simulink model "sf_aircraft_with_empty_monitor"  (R2018a)
settings: Solver=ode4  StartTime=0.0  StopTime=10  RelTol=1e-3  EnableMultiTasking=on
PreLoadFcn:
  | noise_factor=1;
  | load sf_aircraft_buses;
undefined symbols (not defined in the file or in its folder): sf_aircraft_ModeType, sigbuilder_block
libraries: simulink x21, sf_aircraft_screen_library x7, simulink_need_slupdate x2
(part 1 of 2)
settings Model: Creator=The MathWorks, Inc.  LastModifiedBy=matlab
settings DataIOCC: LimitDataPoints=on  SaveFormat=Array  ReturnWorkspaceOutputs=on  SignalLoggingName=sigsOut
settings OptimizationCC: ExpressionDepthLimit=2147483647  InitFltsAndDblsToZero=on  LifeSpan=inf
settings DebuggingCC: SaveWithParameterizedLinksMsg=none  UnderspecifiedInitializationDetection=Classic  MergeDetectMultiDrivingBlocksExec=none  CheckExecutionContextPreStartOutputMsg=on  CheckExecutionContextRuntimeOutputMsg=on  SignalResolutionControl=TryResolveAllWithWarning  MultiTaskDSMMsg=warning  MultiTaskCondExecSysMsg=none  FcnCallInpInsideContextMsg=warning  StateNameClashWarn=warning  SFUnexpectedBacktrackingDiag=warning  SFNoUnconditionalDefaultTransitionDiag=warning  SFExecutionAtInitializationDiag=none
settings HardwareCC: ProdBitPerPointer=32  ProdBitPerSizeT=32  ProdBitPerPtrDiffT=32  ProdLargestAtomicFloat=None  ProdIntDivRoundTo=Undefined  ProdEndianess=Unspecified  ProdWordSize=32  ProdHWDeviceType=32-bit Generic Real Time Simulator
settings ModelReferenceCC: PropagateSignalLabelsOutOfModel=off
settings SFSimCC: SimCustomHeaderCode="#include \"sf_aircraft_ModeType.h\""  SimParseCustomCode=off
settings RTWCC: GenCodeOnly=on  Description=Generic Real-Time Target  GenerateReport=on  CustomHeaderCode="#include \"sf_aircraft_ModeType.h\""
settings CodeAppCC: StateflowObjectComments=on
settings GRTTargetCC: TargetLangStandard=C89/C90 (ANSI)  GeneratePreprocessorConditionals=Disable all
settings ConfigComp: CovMetricSettings=dw  CovHtmlReporting=on  CovSaveCumulativeToWorkspaceVar=on  CovSaveSingleToWorkspaceVar=on  CovExternalEMLEnable=off  CovSFcnEnable=off

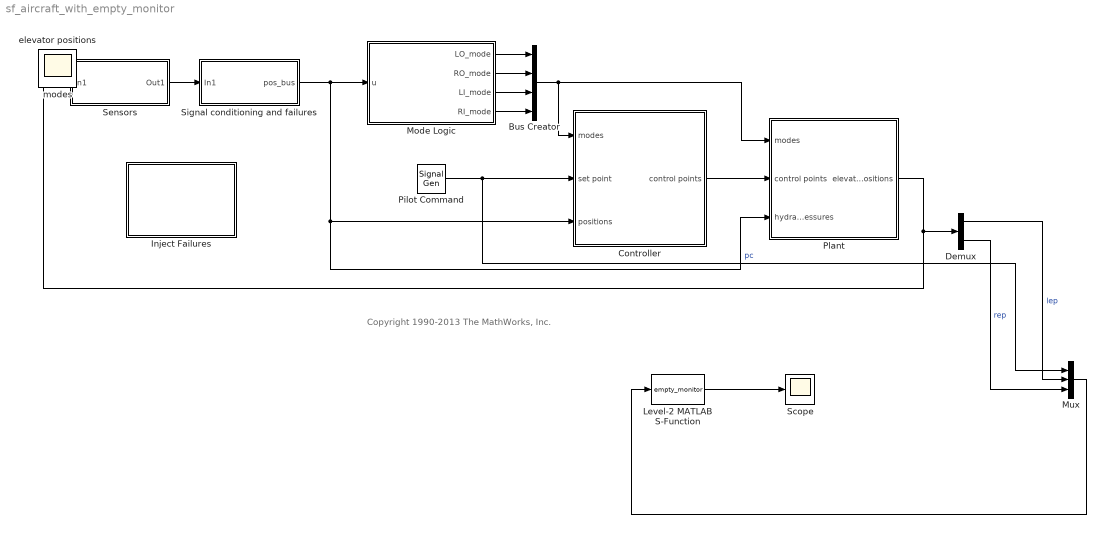
== system sf_aircraft_with_empty_monitor ==
  note: Copyright 1990-2013 The MathWorks, Inc.
  Bus Creator : BusCreator  Inputs=4
  Controller : Subsystem
  Demux : Demux  Outputs=2
  Inject Failures : Subsystem
      settings: OpenFcn=sf_aircraft_failures
      mask Display: disp('Inject Failures GUI')
  Level-2 MATLAB S-Function : M-S-Function  FunctionName=empty_monitor
  Mode Logic : Stateflow chart  TreatAsAtomicUnit=on
  Mux : Mux  Inputs=3
  Pilot Command : SignalGenerator  WaveForm=square  Frequency=0.2
  Plant : Subsystem
      mask Display: image('sf_aircraft_airplane.jpg')
  Scope : Scope
  Sensors : Subsystem
  "Signal conditioning and failures " : Subsystem
  elevator positions : Scope
  modes : Scope
  wires:
  "Signal conditioning and failures "/1(pos_bus) -> Controller/3(positions), Plant/3(hydraulic pressures), Mode Logic/1(u)
  Controller/1(control points) -> Plant/2(control points)
  Pilot Command/1 -> Mux/1, Controller/2(set point)  "pc"
  Sensors/1(Out1) -> "Signal conditioning and failures "/1(In1)
  Bus Creator/1 -> Plant/1(modes), Controller/1(modes)
  Mode Logic/1(" LO_mode") -> Bus Creator/1
  Mode Logic/2(" RO_mode") -> Bus Creator/2
  Mode Logic/3(" LI_mode") -> Bus Creator/3
  Mode Logic/4(" RI_mode") -> Bus Creator/4
  Plant/1(elevator positions) -> Demux/1, Sensors/1(In1)
  Demux/1 -> Mux/2  "lep"
  Demux/2 -> Mux/3  "rep"
  Mux/1 -> Level-2 MATLAB S-Function/1
  Level-2 MATLAB S-Function/1 -> Scope/1

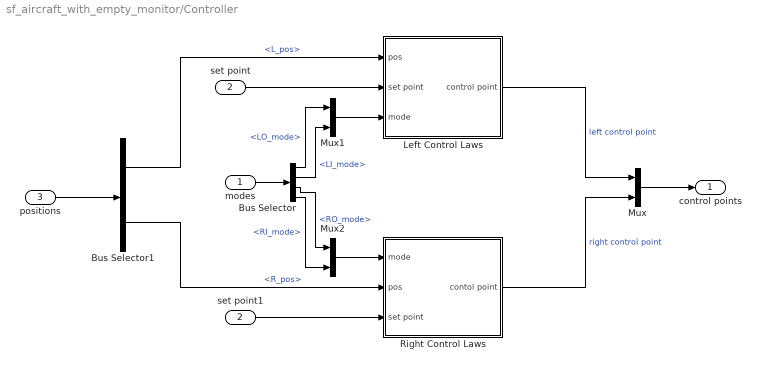
== system sf_aircraft_with_empty_monitor/Controller ==
  modes : Inport
  set point : Inport  Port=2  SampleTime=0.01
  positions : Inport  Port=3  SampleTime=0.01
  Bus Selector : BusSelector  OutputSignals=LO_mode,LI_mode,RO_mode,RI_mode
  Bus Selector1 : BusSelector  OutputSignals=L_pos,R_pos
  Left Control Laws : Subsystem
  Mux : Mux  Inputs=2
  Mux1 : Mux  Inputs=2
  Mux2 : Mux  Inputs=2
  Right Control Laws : Subsystem
  set point1 : InportShadow  Port=2  SampleTime=0.01
  control points : Outport
  wires:
  Mux/1 -> control points/1
  modes/1 -> Bus Selector/1
  Right Control Laws/1(contol point) -> Mux/2  "right control point"
  set point1/1 -> Right Control Laws/3(set point)
  Left Control Laws/1(control point) -> Mux/1  "left control point"
  set point/1 -> Left Control Laws/2(set point)
  Bus Selector/4 -> Mux2/2  "<RI_mode>"
  Bus Selector/3 -> Mux2/1  "<RO_mode>"
  Bus Selector/1 -> Mux1/1  "<LO_mode>"
  Bus Selector/2 -> Mux1/2  "<LI_mode>"
  Mux1/1 -> Left Control Laws/3(mode)
  Mux2/1 -> Right Control Laws/1(mode)
  positions/1 -> Bus Selector1/1
  Bus Selector1/1 -> Left Control Laws/1(pos)  "<L_pos>"
  Bus Selector1/2 -> Right Control Laws/2(pos)  "<R_pos>"

== system sf_aircraft_with_empty_monitor/Inject Failures ==

== system sf_aircraft_with_empty_monitor/Plant ==
  modes : Inport
  control points : Inport  Port=2  SampleTime=0.01
  hydraulic pressures : Inport  Port=3  SampleTime=0.01
  Actuators : Subsystem
  Left Elevator : Subsystem
  Mux : Mux  Inputs=2
  Mux1 : Mux  Inputs=2
  Right Elevator : Subsystem
  elevator positions : Outport
  wires:
  Mux1/1 -> elevator positions/1
  Right Elevator/2(elevator position) -> Mux1/2
  Left Elevator/1(elevator position) -> Mux1/1
  Mux/1 -> Actuators/4(piston velocity)
  Right Elevator/1(elevator velocity) -> Mux/2
  Left Elevator/2(elevator velocity) -> Mux/1
  modes/1 -> Actuators/3(modes)
  Actuators/2(Right piston force) -> Right Elevator/1(piston force)
  hydraulic pressures/1 -> Actuators/2(hydraulic pressure)
  control points/1 -> Actuators/1(control point)
  Actuators/1(Left piston force) -> Left Elevator/1(piston force)

== system sf_aircraft_with_empty_monitor/Sensors ==
  In1 : Inport
  Demux : Demux  Outputs=2
  Measured Left Inner Actuator positions : Subsystem
  Measured Left Outer Actuator positions : Subsystem
  Measured Right Inner Actuator positions : Subsystem
  Measured Right Outer Actuator positions : Subsystem
  Mux : Mux
  Out1 : Outport
  wires:
  Demux/1 -> Measured Left Inner Actuator positions/1(In1), Measured Left Outer Actuator positions/1(In1)
  Demux/2 -> Measured Right Inner Actuator positions/1(In1), Measured Right Outer Actuator positions/1(In1)
  Measured Left Outer Actuator positions/1(Out) -> Mux/1
  Measured Left Inner Actuator positions/1(Out) -> Mux/2
  Measured Right Inner Actuator positions/1(Out) -> Mux/3
  Measured Right Outer Actuator positions/1(Out) -> Mux/4
  In1/1 -> Demux/1
  Mux/1 -> Out1/1

== system sf_aircraft_with_empty_monitor/Signal conditioning and failures  ==
  note: These could be 2/4 separate processors, and typically are not residing on the PFCUs
  In1 : Inport
  Actuator Positions : Subsystem
  Bus Creator1 : BusCreator  Inputs=8  OutDataTypeStr=Bus: PositionBus  NonVirtualBus=on
  Demux : Demux
  Hydraulic Pressures : Subsystem
  pos_bus : Outport
  wires:
  Bus Creator1/1 -> pos_bus/1
  Actuator Positions/2(L_pos_fail) -> Bus Creator1/2  "L_pos_fail"
  Actuator Positions/3(R_pos) -> Bus Creator1/3  "R_pos"
  Actuator Positions/4(R_pos_fail) -> Bus Creator1/4  "R_pos_fail"
  In1/1 -> Demux/1
  Demux/1 -> Actuator Positions/1(Left Outer)
  Demux/2 -> Actuator Positions/2(Left Inner)
  Actuator Positions/1(L_pos) -> Bus Creator1/1  "L_pos"
  Demux/3 -> Actuator Positions/3(Right Inner)
  Demux/4 -> Actuator Positions/4(Right Outer)
  Hydraulic Pressures/1(H1_press) -> Bus Creator1/5  "H1_press"
  Hydraulic Pressures/2(H2_press) -> Bus Creator1/6  "H2_press"
  Hydraulic Pressures/3(H3_press) -> Bus Creator1/7  "H3_press"
  Hydraulic Pressures/4(low_press) -> Bus Creator1/8  "low_press"

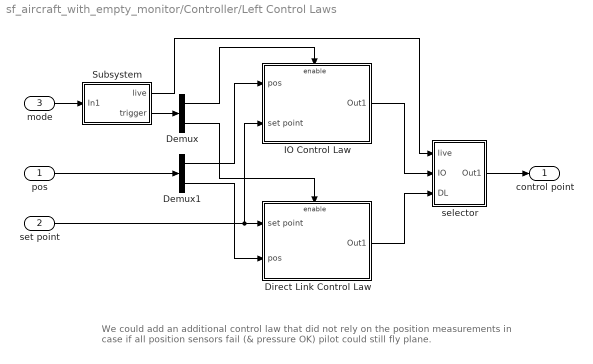
== system sf_aircraft_with_empty_monitor/Controller/Left Control Laws ==
  note: We could add an additional control law that did not rely on the position measurements
      | in case if all position sensors fail (& pressure OK) pilot could still fly plane.
  pos : Inport
  set point : Inport  Port=2  SampleTime=0.01
  mode : Inport  Port=3
  Demux : Demux  Outputs=2
  Demux1 : Demux  Outputs=2
  Direct Link Control Law : Subsystem
  IO Control Law : Subsystem
  Subsystem : Subsystem
  selector : Subsystem
  control point : Outport
  wires:
  Subsystem/1(live) -> selector/1(live)
  set point/1 -> IO Control Law/2(set point), Direct Link Control Law/1(set point)
  pos/1 -> Demux1/1
  selector/1(Out1) -> control point/1
  Direct Link Control Law/1(Out1) -> selector/3(DL)
  IO Control Law/1(Out1) -> selector/2(IO)
  Demux/2 -> Direct Link Control Law/Enable
  Demux/1 -> IO Control Law/Enable
  Subsystem/2(trigger) -> Demux/1
  mode/1 -> Subsystem/1(In1)
  Demux1/1 -> IO Control Law/1(pos)
  Demux1/2 -> Direct Link Control Law/2(pos)

== system sf_aircraft_with_empty_monitor/Controller/Right Control Laws ==
  note: We could add an additional control law that did not have to rely on the position measurements
      | in case if all position sensors fail (& pressure OK) pilot could still fly plane.
  mode : Inport
  pos : Inport  Port=2
  set point : Inport  Port=3  SampleTime=0.01
  Demux : Demux  Outputs=2
  Demux1 : Demux  Outputs=2
  Direct Link Control Law : Subsystem
  IO Control Law : Subsystem
  Subsystem : Subsystem
  selector : Subsystem
  contol point : Outport
  wires:
  selector/1(Out1) -> contol point/1
  Subsystem/1(live) -> selector/1(live)
  Demux1/1 -> IO Control Law/1(pos)
  Demux1/2 -> Direct Link Control Law/2(pos)
  set point/1 -> IO Control Law/2(set point), Direct Link Control Law/1(set point)
  pos/1 -> Demux1/1
  Direct Link Control Law/1(Out1) -> selector/3(DL)
  IO Control Law/1(Out1) -> selector/2(IO)
  Demux/2 -> Direct Link Control Law/Enable
  Demux/1 -> IO Control Law/Enable
  Subsystem/2(trigger) -> Demux/1
  mode/1 -> Subsystem/1(In1)

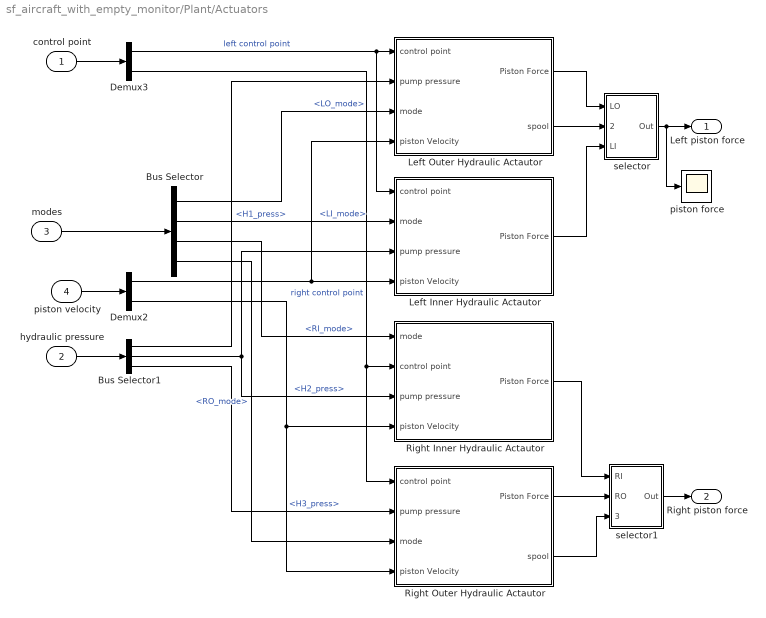
== system sf_aircraft_with_empty_monitor/Plant/Actuators ==
  control point : Inport
  hydraulic pressure : Inport  Port=2
  modes : Inport  Port=3
  piston velocity : Inport  Port=4
  Bus Selector : BusSelector  OutputSignals=LO_mode,LI_mode,RI_mode,RO_mode
  Bus Selector1 : BusSelector  OutputSignals=H1_press,H2_press,H3_press
  Demux2 : Demux  Outputs=2
  Demux3 : Demux  Outputs=2
  Left Inner Hydraulic Actautor : Subsystem
  Left Outer Hydraulic Actautor : Subsystem
  Right Inner Hydraulic Actautor : Subsystem
  Right Outer Hydraulic Actautor : Subsystem
  piston force : Scope
  selector : Subsystem
  selector1 : Subsystem
  Left piston force : Outport
  Right piston force : Outport  Port=2
  wires:
  Right Outer Hydraulic Actautor/2(spool) -> selector1/3(spool)
  Left Outer Hydraulic Actautor/2(spool) -> selector/2(spool)
  Demux3/2 -> Right Outer Hydraulic Actautor/1(control point), Right Inner Hydraulic Actautor/2(control point)  "right control point"
  control point/1 -> Demux3/1
  piston velocity/1 -> Demux2/1
  Demux2/2 -> Right Outer Hydraulic Actautor/4(piston Velocity), Right Inner Hydraulic Actautor/4(piston Velocity)
  modes/1 -> Bus Selector/1
  Bus Selector1/3 -> Right Outer Hydraulic Actautor/2(pump pressure)  "<H3_press>"
  Bus Selector1/2 -> Right Inner Hydraulic Actautor/3(pump pressure), Left Inner Hydraulic Actautor/3(pump pressure)  "<H2_press>"
  selector1/1(Out) -> Right piston force/1
  selector/1(Out) -> Left piston force/1, piston force/1
  Left Inner Hydraulic Actautor/1(Piston Force) -> selector/3(LI)
  Left Outer Hydraulic Actautor/1(Piston Force) -> selector/1(LO)
  Right Outer Hydraulic Actautor/1(Piston Force) -> selector1/2(RO)
  Right Inner Hydraulic Actautor/1(Piston Force) -> selector1/1(RI)
  Demux2/1 -> Left Outer Hydraulic Actautor/4(piston Velocity), Left Inner Hydraulic Actautor/4(piston Velocity)
  Demux3/1 -> Left Inner Hydraulic Actautor/1(control point), Left Outer Hydraulic Actautor/1(control point)  "left control point"
  Bus Selector1/1 -> Left Outer Hydraulic Actautor/2(pump pressure)  "<H1_press>"
  Bus Selector/1 -> Left Outer Hydraulic Actautor/3(mode)  "<LO_mode>"
  Bus Selector/2 -> Left Inner Hydraulic Actautor/2(mode)  "<LI_mode>"
  Bus Selector/3 -> Right Inner Hydraulic Actautor/1(mode)  "<RI_mode>"
  Bus Selector/4 -> Right Outer Hydraulic Actautor/3(mode)  "<RO_mode>"
  hydraulic pressure/1 -> Bus Selector1/1

== system sf_aircraft_with_empty_monitor/Plant/Left Elevator ==
  piston force : Inport
  Sum1 : Sum  Inputs=-+-  SaturateOnIntegerOverflow=on
  elevator Mass : Integrator
  integrator : Integrator
  viscous friction : Gain  Gain=10  SaturateOnIntegerOverflow=on  OutDataTypeStr=Inherit: Same as input  ParamDataTypeStr=Inherit: Same as input
  wind load : Gain  Gain=1000  SaturateOnIntegerOverflow=on  OutDataTypeStr=Inherit: Same as input  ParamDataTypeStr=Inherit: Same as input
  elevator position : Outport
  elevator velocity : Outport  Port=2
  wires:
  Sum1/1 -> elevator Mass/1
  elevator Mass/1 -> viscous friction/1, elevator velocity/1, integrator/1
  integrator/1 -> elevator position/1, wind load/1
  piston force/1 -> Sum1/2
  viscous friction/1 -> Sum1/3
  wind load/1 -> Sum1/1

== system sf_aircraft_with_empty_monitor/Plant/Right Elevator ==
  piston force : Inport
  Sum1 : Sum  Inputs=-+-  SaturateOnIntegerOverflow=on
  elevator Mass : Integrator
  integrator : Integrator
  viscous friction : Gain  Gain=10  SaturateOnIntegerOverflow=on  OutDataTypeStr=Inherit: Same as input  ParamDataTypeStr=Inherit: Same as input
  wind load : Gain  Gain=1000  SaturateOnIntegerOverflow=on  OutDataTypeStr=Inherit: Same as input  ParamDataTypeStr=Inherit: Same as input
  elevator velocity : Outport
  elevator position : Outport  Port=2
  wires:
  integrator/1 -> elevator position/1, wind load/1
  elevator Mass/1 -> integrator/1, viscous friction/1, elevator velocity/1
  Sum1/1 -> elevator Mass/1
  wind load/1 -> Sum1/1
  viscous friction/1 -> Sum1/3
  piston force/1 -> Sum1/2

== system sf_aircraft_with_empty_monitor/Sensors/Measured Left Inner Actuator positions ==
  In1 : Inport
  LI_pos_fail : Constant  Value=0  OutDataTypeStr=boolean
  Measured Position1 : Subsystem
  Measured Position2 : Subsystem
  Measured Position3 : Subsystem
  Mux : Mux  Inputs=3
  Outlier/failure : Subsystem  Tag=STV Subsys  LoadFcn=sigbuilder_block('load');  StartFcn=sigbuilder_block('start');  StopFcn=sigbuilder_block('stop');  ClipboardFcn=sigbuilder_block('clipboard');  mask(Sigbuilder block){tuvar=[0:10]}
      mask help: Sigbuilder GUI
      mask init:
      | if ~strcmp(get_param(bdroot,'SimulationStatus'),'stopped') tuvar = sigbuilder_block('maskInit'); end
      settings: CopyFcn=sigbuilder_block('copy');  DeleteFcn=sigbuilder_block('delete');  ModelCloseFcn=sigbuilder_block('modelClose');  PreSaveFcn=sigbuilder_block('preSave');  PauseFcn=sigbuilder_block('pause')  ContinueFcn=sigbuilder_block('continue')  NameChangeFcn=sigbuilder_block('namechange');  OpenFcn=sigbuilder_block('open',[81 97.5 519.75 399.75 ]);  CloseFcn=sigbuilder_block('close');
      mask Display: plot(0, 0, 100, 100,[2, 2, 32, 32, 2], [68, 8, 8, 68, 68],[32, 2], [38, 38], [32, 19, 2],[53, 60, 44], [32, 17, 17, 2],[16, 16, 31, 31]);txt = getActiveGroup(gcbh);text(2, 100, txt,'verticalAlignment', 'top');
  Switch : Switch  Criteria=u2 ~= 0  SaturateOnIntegerOverflow=on
  Zero-Order Hold : ZeroOrderHold  SampleTime=0.01
  Out : Outport
  wires:
  Switch/1 -> Zero-Order Hold/1
  Measured Position1/1(Out1) -> Mux/1
  Measured Position2/1(Out1) -> Mux/2
  Mux/1 -> Out/1
  Measured Position3/1(Out1) -> Mux/3
  Outlier/failure/1(Signal 1) -> Switch/1
  LI_pos_fail/1 -> Switch/2
  In1/1 -> Switch/3
  Zero-Order Hold/1 -> Measured Position3/1(position), Measured Position1/1(position), Measured Position2/1(position)

== system sf_aircraft_with_empty_monitor/Sensors/Measured Left Outer Actuator positions ==
  In1 : Inport
  LO_pos_fail : Constant  Value=0  OutDataTypeStr=boolean
  Measured Position1 : Subsystem
  Measured Position2 : Subsystem
  Measured Position3 : Subsystem
  Mux : Mux  Inputs=3
  Outlier/failure : Subsystem  Tag=STV Subsys  LoadFcn=sigbuilder_block('load');  StartFcn=sigbuilder_block('start');  StopFcn=sigbuilder_block('stop');  ClipboardFcn=sigbuilder_block('clipboard');  mask(Sigbuilder block){tuvar=[0:10]}
      mask help: Sigbuilder GUI
      mask init:
      | if ~strcmp(get_param(bdroot,'SimulationStatus'),'stopped') tuvar = sigbuilder_block('maskInit'); end
      settings: CopyFcn=sigbuilder_block('copy');  DeleteFcn=sigbuilder_block('delete');  ModelCloseFcn=sigbuilder_block('modelClose');  PreSaveFcn=sigbuilder_block('preSave');  PauseFcn=sigbuilder_block('pause')  ContinueFcn=sigbuilder_block('continue')  NameChangeFcn=sigbuilder_block('namechange');  OpenFcn=sigbuilder_block('open',[81 97.5 519.75 399.75 ]);  CloseFcn=sigbuilder_block('close');
      mask Display: plot(0, 0, 100, 100,[2, 2, 32, 32, 2], [68, 8, 8, 68, 68],[32, 2], [38, 38], [32, 19, 2],[53, 60, 44], [32, 17, 17, 2],[16, 16, 31, 31]);txt = getActiveGroup(gcbh);text(2, 100, txt,'verticalAlignment', 'top');
  Switch : Switch  Criteria=u2 ~= 0  SaturateOnIntegerOverflow=on
  Zero-Order Hold : ZeroOrderHold  SampleTime=0.01
  Out : Outport
  wires:
  Measured Position3/1(Out1) -> Mux/3
  Mux/1 -> Out/1
  Measured Position2/1(Out1) -> Mux/2
  Measured Position1/1(Out1) -> Mux/1
  Switch/1 -> Zero-Order Hold/1
  Outlier/failure/1(Signal 1) -> Switch/1
  LO_pos_fail/1 -> Switch/2
  In1/1 -> Switch/3
  Zero-Order Hold/1 -> Measured Position2/1(position), Measured Position1/1(position), Measured Position3/1(position)

== system sf_aircraft_with_empty_monitor/Sensors/Measured Right Inner Actuator positions ==
  In1 : Inport
  Measured Position1 : Subsystem
  Measured Position2 : Subsystem
  Measured Position3 : Subsystem
  Mux : Mux  Inputs=3
  Outlier/failure : Subsystem  Tag=STV Subsys  LoadFcn=sigbuilder_block('load');  StartFcn=sigbuilder_block('start');  StopFcn=sigbuilder_block('stop');  ClipboardFcn=sigbuilder_block('clipboard');  mask(Sigbuilder block){tuvar=[0:10]}
      mask help: Sigbuilder GUI
      mask init:
      | if ~strcmp(get_param(bdroot,'SimulationStatus'),'stopped') tuvar = sigbuilder_block('maskInit'); end
      settings: CopyFcn=sigbuilder_block('copy');  DeleteFcn=sigbuilder_block('delete');  ModelCloseFcn=sigbuilder_block('modelClose');  PreSaveFcn=sigbuilder_block('preSave');  PauseFcn=sigbuilder_block('pause')  ContinueFcn=sigbuilder_block('continue')  NameChangeFcn=sigbuilder_block('namechange');  OpenFcn=sigbuilder_block('open',[81 97.5 519.75 399.75 ]);  CloseFcn=sigbuilder_block('close');
      mask Display: plot(0, 0, 100, 100,[2, 2, 32, 32, 2], [68, 8, 8, 68, 68],[32, 2], [38, 38], [32, 19, 2],[53, 60, 44], [32, 17, 17, 2],[16, 16, 31, 31]);txt = getActiveGroup(gcbh);text(2, 100, txt,'verticalAlignment', 'top');
  RI_pos_fail : Constant  Value=0  OutDataTypeStr=boolean
  Switch : Switch  Criteria=u2 ~= 0  SaturateOnIntegerOverflow=on
  Zero-Order Hold : ZeroOrderHold  SampleTime=0.01
  Out : Outport
  wires:
  Switch/1 -> Zero-Order Hold/1
  Measured Position1/1(Out1) -> Mux/1
  Measured Position2/1(Out1) -> Mux/2
  Mux/1 -> Out/1
  Measured Position3/1(Out1) -> Mux/3
  Outlier/failure/1(Signal 1) -> Switch/1
  RI_pos_fail/1 -> Switch/2
  In1/1 -> Switch/3
  Zero-Order Hold/1 -> Measured Position3/1(position), Measured Position1/1(position), Measured Position2/1(position)

== system sf_aircraft_with_empty_monitor/Sensors/Measured Right Outer Actuator positions ==
  In1 : Inport
  Measured Position1 : Subsystem
  Measured Position2 : Subsystem
  Measured Position3 : Subsystem
  Mux : Mux  Inputs=3
  Outlier/failure : Subsystem  Tag=STV Subsys  LoadFcn=sigbuilder_block('load');  StartFcn=sigbuilder_block('start');  StopFcn=sigbuilder_block('stop');  ClipboardFcn=sigbuilder_block('clipboard');  mask(Sigbuilder block){tuvar=[0:10]}
      mask help: Sigbuilder GUI
      mask init:
      | if ~strcmp(get_param(bdroot,'SimulationStatus'),'stopped') tuvar = sigbuilder_block('maskInit'); end
      settings: CopyFcn=sigbuilder_block('copy');  DeleteFcn=sigbuilder_block('delete');  ModelCloseFcn=sigbuilder_block('modelClose');  PreSaveFcn=sigbuilder_block('preSave');  PauseFcn=sigbuilder_block('pause')  ContinueFcn=sigbuilder_block('continue')  NameChangeFcn=sigbuilder_block('namechange');  OpenFcn=sigbuilder_block('open',[81 97.5 519.75 399.75 ]);  CloseFcn=sigbuilder_block('close');
      mask Display: plot(0, 0, 100, 100,[2, 2, 32, 32, 2], [68, 8, 8, 68, 68],[32, 2], [38, 38], [32, 19, 2],[53, 60, 44], [32, 17, 17, 2],[16, 16, 31, 31]);txt = getActiveGroup(gcbh);text(2, 100, txt,'verticalAlignment', 'top');
  RO_pos_fail : Constant  Value=0  OutDataTypeStr=boolean
  Switch : Switch  Criteria=u2 ~= 0  SaturateOnIntegerOverflow=on
  Zero-Order Hold : ZeroOrderHold  SampleTime=0.01
  Out : Outport
  wires:
  Zero-Order Hold/1 -> Measured Position2/1(position), Measured Position1/1(position), Measured Position3/1(position)
  In1/1 -> Switch/3
  RO_pos_fail/1 -> Switch/2
  Outlier/failure/1(Signal 1) -> Switch/1
  Measured Position3/1(Out1) -> Mux/3
  Mux/1 -> Out/1
  Measured Position2/1(Out1) -> Mux/2
  Measured Position1/1(Out1) -> Mux/1
  Switch/1 -> Zero-Order Hold/1

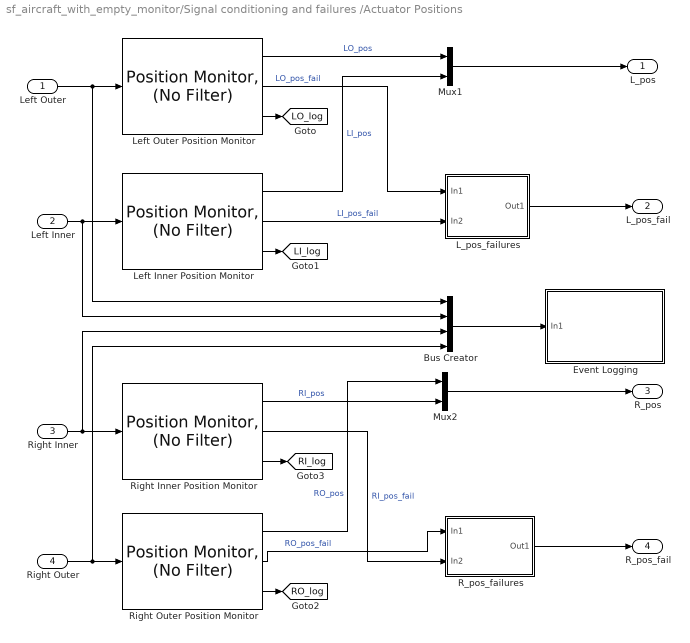
== system sf_aircraft_with_empty_monitor/Signal conditioning and failures /Actuator Positions ==
  Left Outer : Inport
  Left Inner : Inport  Port=2
  Right Inner : Inport  Port=3
  Right Outer : Inport  Port=4
  Bus Creator : BusCreator  Inputs=4
  Event Logging : Subsystem
  L_pos_failures : Subsystem
  Left Inner Position Monitor : sf_aircraft_screen_library/Position Monitor, (No Filter)
      settings: SourceProductName=Stateflow  SourceProductBaseCode=SF
  Left Outer Position Monitor : sf_aircraft_screen_library/Position Monitor, (No Filter)
      settings: SourceProductName=Stateflow  SourceProductBaseCode=SF
  Mux1 : Mux  Inputs=2
  Mux2 : Mux  Inputs=2
  R_pos_failures : Subsystem
  Right Inner Position Monitor : sf_aircraft_screen_library/Position Monitor, (No Filter)
      settings: SourceProductName=Stateflow  SourceProductBaseCode=SF
  Right Outer Position Monitor : sf_aircraft_screen_library/Position Monitor, (No Filter)
      settings: SourceProductName=Stateflow  SourceProductBaseCode=SF
  L_pos : Outport
  L_pos_fail : Outport  Port=2
  R_pos : Outport  Port=3
  R_pos_fail : Outport  Port=4
  tag scope: LI_log=global, LO_log=global, RI_log=global, RO_log=global
  wires:
  Left Outer/1 -> Bus Creator/1, Left Outer Position Monitor/1
  Left Inner/1 -> Bus Creator/2, Left Inner Position Monitor/1
  Left Outer Position Monitor/1 -> Mux1/1  "LO_pos"
  Right Inner/1 -> Bus Creator/3, Right Inner Position Monitor/1
  Right Outer/1 -> Bus Creator/4, Right Outer Position Monitor/1
  Left Inner Position Monitor/1 -> Mux1/2  "LI_pos"
  Left Inner Position Monitor/2 -> L_pos_failures/2(In2)  "LI_pos_fail"
  Right Outer Position Monitor/1 -> Mux2/1  "RO_pos"
  Right Inner Position Monitor/1 -> Mux2/2  "RI_pos"
  Bus Creator/1 -> Event Logging/1(In1)
  Left Outer Position Monitor/3 -> [LO_log]
  Left Inner Position Monitor/3 -> [LI_log]
  Right Outer Position Monitor/3 -> [RO_log]
  Right Inner Position Monitor/3 -> [RI_log]
  Left Outer Position Monitor/2 -> L_pos_failures/1(In1)  "LO_pos_fail"
  Mux1/1 -> L_pos/1
  Mux2/1 -> R_pos/1
  R_pos_failures/1(Out1) -> R_pos_fail/1
  L_pos_failures/1(Out1) -> L_pos_fail/1
  Right Inner Position Monitor/2 -> R_pos_failures/2(In2)  "RI_pos_fail"
  Right Outer Position Monitor/2 -> R_pos_failures/1(In1)  "RO_pos_fail"

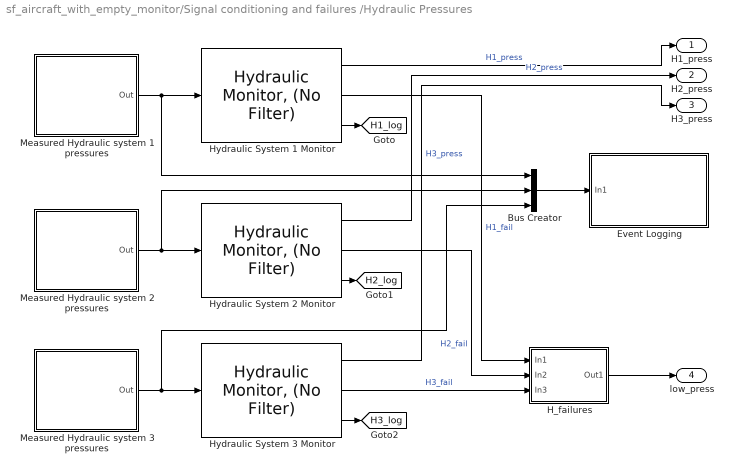
== system sf_aircraft_with_empty_monitor/Signal conditioning and failures /Hydraulic Pressures ==
  Bus Creator : BusCreator  Inputs=3
  Event Logging : Subsystem
  H_failures : Subsystem
  Hydraulic System 1 Monitor : sf_aircraft_screen_library/Hydraulic Monitor, (No Filter)
      settings: SourceProductName=Stateflow  SourceProductBaseCode=SF
  Hydraulic System 2 Monitor : sf_aircraft_screen_library/Hydraulic Monitor, (No Filter)
      settings: SourceProductName=Stateflow  SourceProductBaseCode=SF
  Hydraulic System 3 Monitor : sf_aircraft_screen_library/Hydraulic Monitor, (No Filter)
      settings: SourceProductName=Stateflow  SourceProductBaseCode=SF
  Measured Hydraulic system 1 pressures : Subsystem
  Measured Hydraulic system 2 pressures : Subsystem
  Measured Hydraulic system 3 pressures : Subsystem
  H1_press : Outport
  H2_press : Outport  Port=2
  H3_press : Outport  Port=3
  low_press : Outport  Port=4
  tag scope: H1_log=global, H2_log=global, H3_log=global
  wires:
  H_failures/1(Out1) -> low_press/1
  Hydraulic System 3 Monitor/1 -> H3_press/1  "H3_press"
  Hydraulic System 3 Monitor/2 -> H_failures/3(In3)  "H3_fail"
  Hydraulic System 2 Monitor/2 -> H_failures/2(In2)  "H2_fail"
  Hydraulic System 1 Monitor/2 -> H_failures/1(In1)  "H1_fail"
  Hydraulic System 2 Monitor/1 -> H2_press/1  "H2_press"
  Measured Hydraulic system 3 pressures/1(Out) -> Bus Creator/3, Hydraulic System 3 Monitor/1
  Hydraulic System 1 Monitor/1 -> H1_press/1  "H1_press"
  Measured Hydraulic system 2 pressures/1(Out) -> Bus Creator/2, Hydraulic System 2 Monitor/1
  Measured Hydraulic system 1 pressures/1(Out) -> Bus Creator/1, Hydraulic System 1 Monitor/1
  Bus Creator/1 -> Event Logging/1(In1)
  Hydraulic System 3 Monitor/3 -> [H3_log]
  Hydraulic System 2 Monitor/3 -> [H2_log]
  Hydraulic System 1 Monitor/3 -> [H1_log]

== system sf_aircraft_with_empty_monitor/Controller/Left Control Laws/Direct Link Control Law ==
  set point : Inport
  pos : Inport  Port=2
  Enable : EnablePort  PropagateVarSize=During execution
  Gain : Gain  Gain=0.000325  SaturateOnIntegerOverflow=on  OutDataTypeStr=Inherit: Same as input  ParamDataTypeStr=Inherit: Same as input
  Sum : Sum  Inputs=+-|  SaturateOnIntegerOverflow=on
  Out1 : Outport  InitialOutput=[0]
  wires:
  set point/1 -> Sum/1
  pos/1 -> Sum/2
  Gain/1 -> Out1/1
  Sum/1 -> Gain/1

== system sf_aircraft_with_empty_monitor/Controller/Left Control Laws/IO Control Law ==
  pos : Inport
  set point : Inport  Port=2
  Enable : EnablePort  StatesWhenEnabling=reset  PropagateVarSize=During execution
  PID Controller : simulink_need_slupdate/PID Controller  P=0.0012  I=5.7e-5  D=2.4e-4
      settings: SourceProductName=Simulink
  Sum : Sum  Inputs=+-|  SaturateOnIntegerOverflow=on
  Out1 : Outport  SampleTime=.01  InitialOutput=[0]
  wires:
  set point/1 -> Sum/1
  pos/1 -> Sum/2
  PID Controller/1 -> Out1/1
  Sum/1 -> PID Controller/1

== system sf_aircraft_with_empty_monitor/Controller/Left Control Laws/Subsystem ==
  In1 : Inport
  Constant : Constant  Value=sf_aircraft_ModeType.Active  OutDataTypeStr=Enum: sf_aircraft_ModeType
  Constant1 : Constant  Value=sf_aircraft_ModeType.Standby  OutDataTypeStr=Enum: sf_aircraft_ModeType
  Demux : Demux  Outputs=2
  Logical Operator : Logic  Operator=OR  AllPortsSameDT=off
  Relational Operator : RelationalOperator  Operator===  RndMeth=Nearest
  Relational Operator1 : RelationalOperator  Operator===  RndMeth=Nearest
  Terminator : Terminator
  live : Outport
  trigger : Outport  Port=2
  wires:
  Demux/2 -> Terminator/1
  Demux/1 -> live/1
  Logical Operator/1 -> trigger/1
  Relational Operator1/1 -> Logical Operator/2
  Relational Operator/1 -> Demux/1, Logical Operator/1
  Constant1/1 -> Relational Operator1/2
  In1/1 -> Relational Operator1/1, Relational Operator/1
  Constant/1 -> Relational Operator/2

== system sf_aircraft_with_empty_monitor/Controller/Left Control Laws/selector ==
  live : Inport
  IO : Inport  Port=2
  DL : Inport  Port=3
  Switch : Switch  Criteria=u2 ~= 0  SaturateOnIntegerOverflow=on
  Out1 : Outport  SampleTime=.01
  wires:
  live/1 -> Switch/2
  DL/1 -> Switch/3
  Switch/1 -> Out1/1
  IO/1 -> Switch/1

== system sf_aircraft_with_empty_monitor/Controller/Right Control Laws/Direct Link Control Law ==
  set point : Inport
  pos : Inport  Port=2
  Enable : EnablePort  PropagateVarSize=During execution
  Gain : Gain  Gain=0.000325  SaturateOnIntegerOverflow=on  OutDataTypeStr=Inherit: Same as input  ParamDataTypeStr=Inherit: Same as input
  Sum : Sum  Inputs=+-|  SaturateOnIntegerOverflow=on
  Out1 : Outport  InitialOutput=[0]
  wires:
  set point/1 -> Sum/1
  pos/1 -> Sum/2
  Gain/1 -> Out1/1
  Sum/1 -> Gain/1

== system sf_aircraft_with_empty_monitor/Controller/Right Control Laws/IO Control Law ==
  pos : Inport
  set point : Inport  Port=2
  Enable : EnablePort  PropagateVarSize=During execution
  PID Controller : simulink_need_slupdate/PID Controller  P=0.0012  I=5.7e-5  D=2.4e-4
      settings: SourceProductName=Simulink
  Sum : Sum  Inputs=+-|  SaturateOnIntegerOverflow=on
  Out1 : Outport  SampleTime=.01  InitialOutput=[0]
  wires:
  set point/1 -> Sum/1
  pos/1 -> Sum/2
  PID Controller/1 -> Out1/1
  Sum/1 -> PID Controller/1

== system sf_aircraft_with_empty_monitor/Controller/Right Control Laws/Subsystem ==
  In1 : Inport
  Constant : Constant  Value=sf_aircraft_ModeType.Active  OutDataTypeStr=Enum: sf_aircraft_ModeType
  Constant1 : Constant  Value=sf_aircraft_ModeType.Standby  OutDataTypeStr=Enum: sf_aircraft_ModeType
  Demux : Demux  Outputs=2
  Logical Operator : Logic  Operator=OR  AllPortsSameDT=off
  Relational Operator : RelationalOperator  Operator===  RndMeth=Nearest
  Relational Operator1 : RelationalOperator  Operator===  RndMeth=Nearest
  Terminator : Terminator
  live : Outport
  trigger : Outport  Port=2
  wires:
  Demux/2 -> Terminator/1
  Demux/1 -> live/1
  Logical Operator/1 -> trigger/1
  Relational Operator1/1 -> Logical Operator/2
  Relational Operator/1 -> Demux/1, Logical Operator/1
  Constant1/1 -> Relational Operator1/2
  In1/1 -> Relational Operator1/1, Relational Operator/1
  Constant/1 -> Relational Operator/2

== system sf_aircraft_with_empty_monitor/Controller/Right Control Laws/selector ==
  live : Inport
  IO : Inport  Port=2
  DL : Inport  Port=3
  Switch : Switch  Criteria=u2 ~= 0  SaturateOnIntegerOverflow=on
  Out1 : Outport
  wires:
  live/1 -> Switch/2
  DL/1 -> Switch/3
  Switch/1 -> Out1/1
  IO/1 -> Switch/1

== system sf_aircraft_with_empty_monitor/Plant/Actuators/Left Inner Hydraulic Actautor ==
  control point : Inport
  mode : Inport  Port=2
  pump pressure : Inport  Port=3
  piston Velocity : Inport  Port=4
  Constant1 : Constant  Value=[0 0 0 1 1;0 0 0 0 1]  VectorParams1D=off  OutDataTypeStr=boolean
  Data Type Conversion : DataTypeConversion
  Demux : Demux  Outputs=2
  Direct Look-Up Table : LookupNDDirect  InputsSelectThisObjectFromTable=Vector  TableIsInput=on  Table=[0 0 1 1;0 0 0 1]  DiagnosticForOutOfRangeInput=Error
  Hydraulic Actuator : Subsystem
  Piston Force : Outport
  wires:
  Hydraulic Actuator/1(Piston Force) -> Piston Force/1
  control point/1 -> Hydraulic Actuator/1(set point)
  Constant1/1 -> Direct Look-Up Table/2
  Direct Look-Up Table/1 -> Demux/1
  Demux/2 -> Hydraulic Actuator/4(spool)
  Demux/1 -> Hydraulic Actuator/3(servo)
  mode/1 -> Data Type Conversion/1
  piston Velocity/1 -> Hydraulic Actuator/5(piston velocity)
  pump pressure/1 -> Hydraulic Actuator/2(pump pressure)
  Data Type Conversion/1 -> Direct Look-Up Table/1

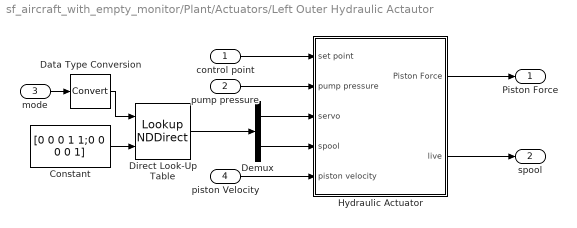
== system sf_aircraft_with_empty_monitor/Plant/Actuators/Left Outer Hydraulic Actautor ==
  control point : Inport
  pump pressure : Inport  Port=2
  mode : Inport  Port=3
  piston Velocity : Inport  Port=4
  Constant : Constant  Value=[0 0 0 1 1;0 0 0 0 1]  VectorParams1D=off  OutDataTypeStr=boolean
  Data Type Conversion : DataTypeConversion
  Demux : Demux  Outputs=2
  Direct Look-Up Table : LookupNDDirect  InputsSelectThisObjectFromTable=Vector  TableIsInput=on  Table=[0 0 1 1;0 0 0 1]  DiagnosticForOutOfRangeInput=Error
  Hydraulic Actuator : Subsystem
  Piston Force : Outport
  spool : Outport  Port=2
  wires:
  Hydraulic Actuator/2(live) -> spool/1
  piston Velocity/1 -> Hydraulic Actuator/5(piston velocity)
  Demux/2 -> Hydraulic Actuator/4(spool)
  Demux/1 -> Hydraulic Actuator/3(servo)
  pump pressure/1 -> Hydraulic Actuator/2(pump pressure)
  control point/1 -> Hydraulic Actuator/1(set point)
  Hydraulic Actuator/1(Piston Force) -> Piston Force/1
  Constant/1 -> Direct Look-Up Table/2
  Direct Look-Up Table/1 -> Demux/1
  mode/1 -> Data Type Conversion/1
  Data Type Conversion/1 -> Direct Look-Up Table/1

== system sf_aircraft_with_empty_monitor/Plant/Actuators/Right Inner Hydraulic Actautor ==
  mode : Inport
  control point : Inport  Port=2
  pump pressure : Inport  Port=3
  piston Velocity : Inport  Port=4
  Constant : Constant  Value=[0 0 0 1 1;0 0 0 0 1]  VectorParams1D=off  OutDataTypeStr=boolean
  Data Type Conversion : DataTypeConversion
  Demux : Demux  Outputs=2
  Direct Look-Up Table : LookupNDDirect  InputsSelectThisObjectFromTable=Vector  TableIsInput=on  Table=[0 0 1 1;0 0 0 1]  DiagnosticForOutOfRangeInput=Error
  Hydraulic Actuator : Subsystem
  Piston Force : Outport
  wires:
  piston Velocity/1 -> Hydraulic Actuator/5(piston velocity)
  Demux/2 -> Hydraulic Actuator/4(spool)
  Demux/1 -> Hydraulic Actuator/3(servo)
  pump pressure/1 -> Hydraulic Actuator/2(pump pressure)
  control point/1 -> Hydraulic Actuator/1(set point)
  Hydraulic Actuator/1(Piston Force) -> Piston Force/1
  Constant/1 -> Direct Look-Up Table/2
  Direct Look-Up Table/1 -> Demux/1
  mode/1 -> Data Type Conversion/1
  Data Type Conversion/1 -> Direct Look-Up Table/1

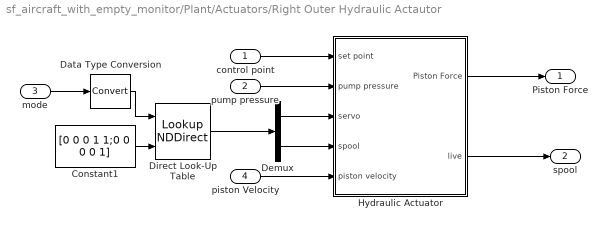
== system sf_aircraft_with_empty_monitor/Plant/Actuators/Right Outer Hydraulic Actautor ==
  control point : Inport
  pump pressure : Inport  Port=2
  mode : Inport  Port=3
  piston Velocity : Inport  Port=4
  Constant1 : Constant  Value=[0 0 0 1 1;0 0 0 0 1]  VectorParams1D=off  OutDataTypeStr=boolean
  Data Type Conversion : DataTypeConversion
  Demux : Demux  Outputs=2
  Direct Look-Up Table : LookupNDDirect  InputsSelectThisObjectFromTable=Vector  TableIsInput=on  Table=[0 0 1 1;0 0 0 1]  DiagnosticForOutOfRangeInput=Error
  Hydraulic Actuator : Subsystem
  Piston Force : Outport
  spool : Outport  Port=2
  wires:
  piston Velocity/1 -> Hydraulic Actuator/5(piston velocity)
  Demux/2 -> Hydraulic Actuator/4(spool)
  Demux/1 -> Hydraulic Actuator/3(servo)
  pump pressure/1 -> Hydraulic Actuator/2(pump pressure)
  control point/1 -> Hydraulic Actuator/1(set point)
  Hydraulic Actuator/2(live) -> spool/1
  Hydraulic Actuator/1(Piston Force) -> Piston Force/1
  Constant1/1 -> Direct Look-Up Table/2
  Direct Look-Up Table/1 -> Demux/1
  mode/1 -> Data Type Conversion/1
  Data Type Conversion/1 -> Direct Look-Up Table/1

== system sf_aircraft_with_empty_monitor/Plant/Actuators/selector ==
  LO : Inport
  spool : Inport  Port=2
  LI : Inport  Port=3
  Switch : Switch  Criteria=u2 ~= 0  SaturateOnIntegerOverflow=on
  Out : Outport
  wires:
  spool/1 -> Switch/2
  LI/1 -> Switch/3
  Switch/1 -> Out/1
  LO/1 -> Switch/1

== system sf_aircraft_with_empty_monitor/Plant/Actuators/selector1 ==
  RI : Inport
  RO : Inport  Port=2
  spool : Inport  Port=3
  Switch : Switch  Criteria=u2 ~= 0  SaturateOnIntegerOverflow=on
  Out : Outport
  wires:
  RO/1 -> Switch/1
  Switch/1 -> Out/1
  RI/1 -> Switch/3
  spool/1 -> Switch/2

== system sf_aircraft_with_empty_monitor/Sensors/Measured Left Inner Actuator positions/Measured Position1 ==
  position : Inport
  Band-Limited White Noise : simulink/Sources/Band-Limited White Noise  Cov=[0.00001]*noise_factor  Ts=0.01  seed=[23651]
  Sum1 : Sum  Inputs=|++  SaturateOnIntegerOverflow=on
  Out1 : Outport
  wires:
  Band-Limited White Noise/1 -> Sum1/2
  position/1 -> Sum1/1
  Sum1/1 -> Out1/1

== system sf_aircraft_with_empty_monitor/Sensors/Measured Left Inner Actuator positions/Measured Position2 ==
  position : Inport
  Band-Limited White Noise : simulink/Sources/Band-Limited White Noise  Cov=[0.00001]*noise_factor  Ts=0.01  seed=[431]
  Sum1 : Sum  Inputs=|++  SaturateOnIntegerOverflow=on
  Out1 : Outport
  wires:
  Sum1/1 -> Out1/1
  position/1 -> Sum1/1
  Band-Limited White Noise/1 -> Sum1/2

== system sf_aircraft_with_empty_monitor/Sensors/Measured Left Inner Actuator positions/Measured Position3 ==
  position : Inport
  Band-Limited White Noise : simulink/Sources/Band-Limited White Noise  Cov=[0.00001]*noise_factor  Ts=0.01  seed=[27423]
  Sum : Sum  Inputs=|++  SaturateOnIntegerOverflow=on
  Out1 : Outport
  wires:
  Band-Limited White Noise/1 -> Sum/2
  position/1 -> Sum/1
  Sum/1 -> Out1/1

== system sf_aircraft_with_empty_monitor/Sensors/Measured Left Inner Actuator positions/Outlier//failure ==
  Demux : Demux  Tag=STV Demux  Outputs=1
  FromWs : FromWorkspace  Tag=STV FromWs  VariableName=tuvar  SampleTime=0
      SigBuilderData=|
      | dataSet.timeRange = [0 30]
      | dataSet.name = 'Group 1'
      | sbobj.Groups.Name = 'Group 1'
      | sbobj.Groups.Signals.Name = 'Signal 1'
      | sbobj.Groups.Signals.XData = [0 30]
      | sbobj.Groups.Signals.YData = [15 15]
      | sbobj.Groups.TimeRange = [0 30]
  Signal 1 : Outport  Tag=STV Outport
  wires:
  FromWs/1 -> Demux/1
  Demux/1 -> Signal 1/1

== system sf_aircraft_with_empty_monitor/Sensors/Measured Left Outer Actuator positions/Measured Position1 ==
  position : Inport
  Band-Limited White Noise : simulink/Sources/Band-Limited White Noise  Cov=[0.00001]*noise_factor  Ts=0.01  seed=[23341]
  Sum1 : Sum  Inputs=|++  SaturateOnIntegerOverflow=on
  Out1 : Outport
  wires:
  Sum1/1 -> Out1/1
  position/1 -> Sum1/1
  Band-Limited White Noise/1 -> Sum1/2

== system sf_aircraft_with_empty_monitor/Sensors/Measured Left Outer Actuator positions/Measured Position2 ==
  position : Inport
  Band-Limited White Noise : simulink/Sources/Band-Limited White Noise  Cov=[0.00001]*noise_factor  Ts=0.01  seed=[1]
  Sum1 : Sum  Inputs=|++  SaturateOnIntegerOverflow=on
  Out1 : Outport
  wires:
  Band-Limited White Noise/1 -> Sum1/2
  position/1 -> Sum1/1
  Sum1/1 -> Out1/1

== system sf_aircraft_with_empty_monitor/Sensors/Measured Left Outer Actuator positions/Measured Position3 ==
  position : Inport
  Band-Limited White Noise : simulink/Sources/Band-Limited White Noise  Cov=[0.00001]*noise_factor  Ts=0.01  seed=[2]
  Sum : Sum  Inputs=|++  SaturateOnIntegerOverflow=on
  Out1 : Outport
  wires:
  Sum/1 -> Out1/1
  position/1 -> Sum/1
  Band-Limited White Noise/1 -> Sum/2

== system sf_aircraft_with_empty_monitor/Sensors/Measured Left Outer Actuator positions/Outlier//failure ==
  Demux : Demux  Tag=STV Demux  Outputs=1
  FromWs : FromWorkspace  Tag=STV FromWs  VariableName=tuvar  SampleTime=0
      SigBuilderData=|
      | dataSet(1).timeRange = [0 30]
      | dataSet(1).name = 'Test 1'
      | dataSet(2).timeRange = [0 30]
      | dataSet(2).name = 'Test 2'
      | sbobj.Groups(1).Name = 'Test 1'
      | sbobj.Groups(1).Signals.Name = 'Signal 1'
      | sbobj.Groups(1).Signals.XData = [0 30]
      | sbobj.Groups(1).Signals.YData = [15 15]
      | sbobj.Groups(1).TimeRange = [0 30]
      | sbobj.Groups(2).Name = 'Test 2'
      | sbobj.Groups(2).Signals.Name = 'Signal 1'
      | sbobj.Groups(2).Signals.XData = [0 30]
      | sbobj.Groups(2).Signals.YData = [15 15]
      | sbobj.Groups(2).TimeRange = [0 30]
  Signal 1 : Outport  Tag=STV Outport
  wires:
  FromWs/1 -> Demux/1
  Demux/1 -> Signal 1/1

== system sf_aircraft_with_empty_monitor/Sensors/Measured Right Inner Actuator positions/Measured Position1 ==
  position : Inport
  Band-Limited White Noise : simulink/Sources/Band-Limited White Noise  Cov=[0.00001]*noise_factor  Ts=0.01  seed=[13651]
  Sum1 : Sum  Inputs=|++  SaturateOnIntegerOverflow=on
  Out1 : Outport
  wires:
  Band-Limited White Noise/1 -> Sum1/2
  position/1 -> Sum1/1
  Sum1/1 -> Out1/1

== system sf_aircraft_with_empty_monitor/Sensors/Measured Right Inner Actuator positions/Measured Position2 ==
  position : Inport
  Band-Limited White Noise : simulink/Sources/Band-Limited White Noise  Cov=[0.00001]*noise_factor  Ts=0.01  seed=[4121]
  Sum1 : Sum  Inputs=|++  SaturateOnIntegerOverflow=on
  Out1 : Outport
  wires:
  Sum1/1 -> Out1/1
  position/1 -> Sum1/1
  Band-Limited White Noise/1 -> Sum1/2

== system sf_aircraft_with_empty_monitor/Sensors/Measured Right Inner Actuator positions/Measured Position3 ==
  position : Inport
  Band-Limited White Noise : simulink/Sources/Band-Limited White Noise  Cov=[0.00001]*noise_factor  Ts=0.01  seed=[4423]
  Sum : Sum  Inputs=|++  SaturateOnIntegerOverflow=on
  Out1 : Outport
  wires:
  Band-Limited White Noise/1 -> Sum/2
  position/1 -> Sum/1
  Sum/1 -> Out1/1

== system sf_aircraft_with_empty_monitor/Sensors/Measured Right Inner Actuator positions/Outlier//failure ==
  Demux : Demux  Tag=STV Demux  Outputs=1
  FromWs : FromWorkspace  Tag=STV FromWs  VariableName=tuvar  SampleTime=0
      SigBuilderData=|
      | dataSet.timeRange = [0 30]
      | dataSet.name = 'Group 1'
      | sbobj.Groups.Name = 'Group 1'
      | sbobj.Groups.Signals.Name = 'Signal 1'
      | sbobj.Groups.Signals.XData = [0 30]
      | sbobj.Groups.Signals.YData = [15 15]
      | sbobj.Groups.TimeRange = [0 30]
  Signal 1 : Outport  Tag=STV Outport
  wires:
  FromWs/1 -> Demux/1
  Demux/1 -> Signal 1/1

== system sf_aircraft_with_empty_monitor/Sensors/Measured Right Outer Actuator positions/Measured Position1 ==
  position : Inport
  Band-Limited White Noise : simulink/Sources/Band-Limited White Noise  Cov=[0.00001]*noise_factor  Ts=0.01  seed=[13651]
  Sum1 : Sum  Inputs=|++  SaturateOnIntegerOverflow=on
  Out1 : Outport
  wires:
  Sum1/1 -> Out1/1
  position/1 -> Sum1/1
  Band-Limited White Noise/1 -> Sum1/2

== system sf_aircraft_with_empty_monitor/Sensors/Measured Right Outer Actuator positions/Measured Position2 ==
  position : Inport
  Band-Limited White Noise : simulink/Sources/Band-Limited White Noise  Cov=[0.00001]*noise_factor  Ts=0.01  seed=[4121]
  Sum1 : Sum  Inputs=|++  SaturateOnIntegerOverflow=on
  Out1 : Outport
  wires:
  Band-Limited White Noise/1 -> Sum1/2
  position/1 -> Sum1/1
  Sum1/1 -> Out1/1

== system sf_aircraft_with_empty_monitor/Sensors/Measured Right Outer Actuator positions/Measured Position3 ==
  position : Inport
  Band-Limited White Noise : simulink/Sources/Band-Limited White Noise  Cov=[0.00001]*noise_factor  Ts=0.01  seed=[4423]
  Sum : Sum  Inputs=|++  SaturateOnIntegerOverflow=on
  Out1 : Outport
  wires:
  Sum/1 -> Out1/1
  position/1 -> Sum/1
  Band-Limited White Noise/1 -> Sum/2

== system sf_aircraft_with_empty_monitor/Sensors/Measured Right Outer Actuator positions/Outlier//failure ==
  Demux : Demux  Tag=STV Demux  Outputs=1
  FromWs : FromWorkspace  Tag=STV FromWs  VariableName=tuvar  SampleTime=0
      SigBuilderData=|
      | dataSet.timeRange = [0 30]
      | dataSet.name = 'Group 1'
      | sbobj.Groups.Name = 'Group 1'
      | sbobj.Groups.Signals.Name = 'Signal 1'
      | sbobj.Groups.Signals.XData = [0 30]
      | sbobj.Groups.Signals.YData = [15 15]
  Signal 1 : Outport  Tag=STV Outport
  wires:
  Demux/1 -> Signal 1/1
  FromWs/1 -> Demux/1

== system sf_aircraft_with_empty_monitor/Signal conditioning and failures /Actuator Positions/Event Logging ==
  In1 : Inport
  Bus Selector : BusSelector  OutputSignals=signal1,signal2,signal3,signal4
  Log LI Actuator Position Sensors : Subsystem  TreatAsAtomicUnit=on
  Log LO Actuator Position Sensors : Subsystem  TreatAsAtomicUnit=on
  Log RI Actuator Position Sensors : Subsystem  TreatAsAtomicUnit=on
  Log RO Actuator Position Sensors : Subsystem  TreatAsAtomicUnit=on
  wires:
  [LO_log] -> Log LO Actuator Position Sensors/Enable
  In1/1 -> Bus Selector/1
  [LI_log] -> Log LI Actuator Position Sensors/Enable
  [RO_log] -> Log RO Actuator Position Sensors/Enable
  [RI_log] -> Log RI Actuator Position Sensors/Enable
  Bus Selector/1 -> Log LO Actuator Position Sensors/1(In1)  "<signal1>"
  Bus Selector/2 -> Log LI Actuator Position Sensors/1(In1)  "<signal2>"
  Bus Selector/3 -> Log RO Actuator Position Sensors/1(In1)  "<signal3>"
  Bus Selector/4 -> Log RI Actuator Position Sensors/1(In1)  "<signal4>"

== system sf_aircraft_with_empty_monitor/Signal conditioning and failures /Actuator Positions/L_pos_failures ==
  In1 : Inport
  In2 : Inport  Port=2
  Mux1 : Mux  Inputs=2
  Out1 : Outport
  wires:
  In1/1 -> Mux1/1
  In2/1 -> Mux1/2
  Mux1/1 -> Out1/1

== system sf_aircraft_with_empty_monitor/Signal conditioning and failures /Actuator Positions/R_pos_failures ==
  In1 : Inport
  In2 : Inport  Port=2
  Mux1 : Mux  Inputs=2
  Out1 : Outport
  wires:
  In1/1 -> Mux1/1
  In2/1 -> Mux1/2
  Mux1/1 -> Out1/1

== system sf_aircraft_with_empty_monitor/Signal conditioning and failures /Hydraulic Pressures/Event Logging ==
  In1 : Inport
  Bus Selector : BusSelector  OutputSignals=signal1,signal2,signal3
  Log Hydraulic System 1 Sensors : Subsystem  TreatAsAtomicUnit=on
  Log Hydraulic System 2 Sensors : Subsystem  TreatAsAtomicUnit=on
  Log Hydraulic System 3 Sensors : Subsystem  TreatAsAtomicUnit=on
  wires:
  [H1_log] -> Log Hydraulic System 1 Sensors/Enable
  In1/1 -> Bus Selector/1
  [H2_log] -> Log Hydraulic System 2 Sensors/Enable
  [H3_log] -> Log Hydraulic System 3 Sensors/Enable
  Bus Selector/1 -> Log Hydraulic System 1 Sensors/1(In1)  "<signal1>"
  Bus Selector/2 -> Log Hydraulic System 2 Sensors/1(In1)  "<signal2>"
  Bus Selector/3 -> Log Hydraulic System 3 Sensors/1(In1)  "<signal3>"

== system sf_aircraft_with_empty_monitor/Signal conditioning and failures /Hydraulic Pressures/H_failures ==
  note: Send to Gauges for Display
  In1 : Inport
  In2 : Inport  Port=2
  In3 : Inport  Port=3
  Mux : Mux  Inputs=3
  Out1 : Outport
  wires:
  In1/1 -> Mux/1
  In2/1 -> Mux/2
  In3/1 -> Mux/3
  Mux/1 -> Out1/1

== system sf_aircraft_with_empty_monitor/Signal conditioning and failures /Hydraulic Pressures/Measured Hydraulic system 1 pressures ==
  Hydraulic pressure : Subsystem
  Mux : Mux  Inputs=3
  pressure reading1 : Subsystem
  pressure reading2 : Subsystem
  pressure reading3 : Subsystem
  Out : Outport
  wires:
  Mux/1 -> Out/1
  pressure reading3/1(Out1) -> Mux/3
  pressure reading2/1(Out1) -> Mux/2
  pressure reading1/1(Out1) -> Mux/1
  Hydraulic pressure/1(Out1) -> pressure reading1/1(pressure), pressure reading2/1(pressure), pressure reading3/1(pressure)

== system sf_aircraft_with_empty_monitor/Signal conditioning and failures /Hydraulic Pressures/Measured Hydraulic system 2 pressures ==
  Hydraulic pressure : Subsystem
  Mux : Mux  Inputs=3
  pressure reading1 : Subsystem
  pressure reading2 : Subsystem
  pressure reading3 : Subsystem
  Out : Outport
  wires:
  Hydraulic pressure/1(Out1) -> pressure reading3/1(pressure), pressure reading2/1(pressure), pressure reading1/1(pressure)
  pressure reading1/1(Out1) -> Mux/1
  pressure reading2/1(Out1) -> Mux/2
  pressure reading3/1(Out1) -> Mux/3
  Mux/1 -> Out/1

== system sf_aircraft_with_empty_monitor/Signal conditioning and failures /Hydraulic Pressures/Measured Hydraulic system 3 pressures ==
  Hydraulic pressure : Subsystem
  Mux : Mux  Inputs=3
  pressure reading1 : Subsystem
  pressure reading2 : Subsystem
  pressure reading3 : Subsystem
  Out : Outport
  wires:
  Mux/1 -> Out/1
  pressure reading3/1(Out1) -> Mux/3
  pressure reading2/1(Out1) -> Mux/2
  pressure reading1/1(Out1) -> Mux/1
  Hydraulic pressure/1(Out1) -> pressure reading1/1(pressure), pressure reading2/1(pressure), pressure reading3/1(pressure)

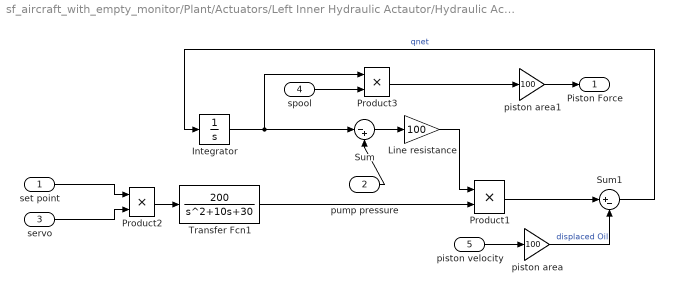
== system sf_aircraft_with_empty_monitor/Plant/Actuators/Left Inner Hydraulic Actautor/Hydraulic Actuator ==
  set point : Inport
  pump pressure : Inport  Port=2
  servo : Inport  Port=3
  spool : Inport  Port=4
  piston velocity : Inport  Port=5
  Integrator : Integrator
  Line resistance : Gain  Gain=100  SaturateOnIntegerOverflow=on  OutDataTypeStr=Inherit: Same as input  ParamDataTypeStr=Inherit: Same as input
  Product1 : Product  SaturateOnIntegerOverflow=on  OutDataTypeStr=Inherit: Same as first input
  Product2 : Product  SaturateOnIntegerOverflow=on  OutDataTypeStr=Inherit: Same as first input
  Product3 : Product  SaturateOnIntegerOverflow=on  OutDataTypeStr=Inherit: Same as first input
  Sum : Sum  Inputs=|-+  SaturateOnIntegerOverflow=on
  Sum1 : Sum  Inputs=|+-  SaturateOnIntegerOverflow=on
  Transfer Fcn1 : TransferFcn  Numerator=[200]  Denominator=[1 10 30]
  piston area : Gain  Gain=100  SaturateOnIntegerOverflow=on  OutDataTypeStr=Inherit: Same as input  ParamDataTypeStr=Inherit: Same as input
  piston area1 : Gain  Gain=100  SaturateOnIntegerOverflow=on  OutDataTypeStr=Inherit: Same as input  ParamDataTypeStr=Inherit: Same as input
  Piston Force : Outport
  wires:
  spool/1 -> Product3/2
  Product3/1 -> piston area1/1
  servo/1 -> Product2/2
  Product2/1 -> Transfer Fcn1/1
  set point/1 -> Product2/1
  piston area1/1 -> Piston Force/1
  pump pressure/1 -> Sum/2
  Integrator/1 -> Sum/1, Product3/1
  Sum1/1 -> Integrator/1  "qnet"
  piston area/1 -> Sum1/2  "displaced Oil"
  piston velocity/1 -> piston area/1
  Product1/1 -> Sum1/1
  Transfer Fcn1/1 -> Product1/2
  Line resistance/1 -> Product1/1
  Sum/1 -> Line resistance/1

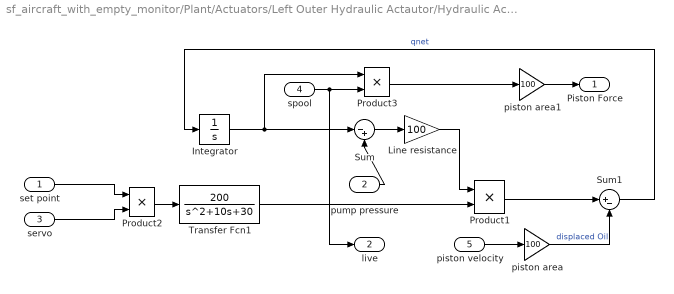
== system sf_aircraft_with_empty_monitor/Plant/Actuators/Left Outer Hydraulic Actautor/Hydraulic Actuator ==
  set point : Inport
  pump pressure : Inport  Port=2
  servo : Inport  Port=3
  spool : Inport  Port=4
  piston velocity : Inport  Port=5
  Integrator : Integrator
  Line resistance : Gain  Gain=100  SaturateOnIntegerOverflow=on  OutDataTypeStr=Inherit: Same as input  ParamDataTypeStr=Inherit: Same as input
  Product1 : Product  SaturateOnIntegerOverflow=on  OutDataTypeStr=Inherit: Same as first input
  Product2 : Product  SaturateOnIntegerOverflow=on  OutDataTypeStr=Inherit: Same as first input
  Product3 : Product  SaturateOnIntegerOverflow=on  OutDataTypeStr=Inherit: Same as first input
  Sum : Sum  Inputs=|-+  SaturateOnIntegerOverflow=on
  Sum1 : Sum  Inputs=|+-  SaturateOnIntegerOverflow=on
  Transfer Fcn1 : TransferFcn  Numerator=[200]  Denominator=[1 10 30]
  piston area : Gain  Gain=100  SaturateOnIntegerOverflow=on  OutDataTypeStr=Inherit: Same as input  ParamDataTypeStr=Inherit: Same as input
  piston area1 : Gain  Gain=100  SaturateOnIntegerOverflow=on  OutDataTypeStr=Inherit: Same as input  ParamDataTypeStr=Inherit: Same as input
  Piston Force : Outport
  live : Outport  Port=2
  wires:
  spool/1 -> live/1, Product3/2
  Product3/1 -> piston area1/1
  servo/1 -> Product2/2
  Product2/1 -> Transfer Fcn1/1
  set point/1 -> Product2/1
  piston area1/1 -> Piston Force/1
  pump pressure/1 -> Sum/2
  Integrator/1 -> Sum/1, Product3/1
  Sum1/1 -> Integrator/1  "qnet"
  piston area/1 -> Sum1/2  "displaced Oil"
  piston velocity/1 -> piston area/1
  Product1/1 -> Sum1/1
  Transfer Fcn1/1 -> Product1/2
  Line resistance/1 -> Product1/1
  Sum/1 -> Line resistance/1
